simulink model "UNIFIER"  (R2023b)
settings: Solver=ode1  StartTime=0.0  StopTime=60  FixedStep=1/500  RelTol=1e-3
values from neighbouring files (symbols this model uses):
  b = 20.11467    [UNIFIER_LOAD.m]
  c = 1.43676    [UNIFIER_LOAD.m]
  DEP_INTEG_IC = 117.49388    [UNIFIER_LOAD.m]
  Euler0 = [3.43106170068520e-06, 0.0515008506277664, -2.79252663434261]    [UNIFIER_LOAD.m]
  ground_alt = 0    [UNIFIER_LOAD.m]
  h_ref_for_xplane = 0    [UNIFIER_LOAD.m]
  m = 7057    [UNIFIER_LOAD.m]
  omegab0 = [0,0,0]    [UNIFIER_LOAD.m]
  S = 29.98388    [UNIFIER_LOAD.m]
  sensor_delay_steps = 5    [UNIFIER_LOAD.m]
  u1_0 = [2.1112539e-05, -2.1112539e-05, -0.085004635, -0.084972650, 0.19720161, 0.19720161]    [UNIFIER_LOAD.m]
  u2_0 = ones(1,12) .* 0.4252    [UNIFIER_LOAD.m]
  u3_0 = 0.089689    [UNIFIER_LOAD.m]
  u4_0 = 0    [UNIFIER_LOAD.m]
  Vb0 = [52.6789583501891, 0, 2.71559652634250]    [UNIFIER_LOAD.m]
  vtail_dist_to_wing = 7.8070    (= 7.807)    [UNIFIER_LOAD.m]
  vtail_nodes = [dp_VTAIL.Xs_LE;     dp_VTAIL.Ys_LE;     dp_VTAIL.Zs_LE]    [UNIFIER_LOAD.m]
  wing_nodes = [fliplr(dp_WING_tip.LE_Xs),fliplr(dp_WING_root.LE_Xs),dp_WING_root.LE_Xs,dp_WING_tip.LE_Xs;     fliplr(-dp_WING_tip.LE_Ys),fliplr(-dp_WING_root.LE_Ys),dp_WING_root.LE_Ys,dp_WING_tip.LE_Ys;     fliplr(dp_WING_tip.LE_Zs),fliplr(dp_WING_root.LE_Zs),dp_WING_root.LE_Zs,dp_WING_tip.LE_Zs]    [UNIFIER_LOAD.m]
  Xe0 = [0,0,-1100]    [UNIFIER_LOAD.m]
  xyz_cg = [-8.09,0,-0.2]    [UNIFIER_LOAD.m]
  xyz_DEP = [ -6.9629998	-6.9210000	-6.8660002	-6.8099999	-6.7540002	-6.6999998	-6.6999998	-6.7540002	-6.8099999	-6.8660002	-6.9210000	-6.9629998 ... (first row only)    [UNIFIER_LOAD.m]
undefined symbols (not defined in the file or in its folder): dp_DEP, dp_FUSE_FIN, dp_HTU, dp_VTAIL, dp_VTAIL_INDUCED, dp_WING_root, dp_WING_tip, Earth, F, fcc, MIL, WGS84
libraries: aerolibactuator x16, dspnetwork x15, sharedutil x14, simulink_extras x13, sharedtransform x7, aerolibtransform2 x5, simulink x5, aerolibwind2 x4, matrix_library x1, shared6dof x1, aerolibatmos2 x1, slpidlib x1
(part 4 of 4)

== system UNIFIER/C7A_HARW/Subsystems/LandingGears/LeftMain/DetermineGroundImpact ==
  X_gear : Inport
  ground_alt : Inport  Port=2
  MATLAB Function : MATLAB Function  TreatAsAtomicUnit=on
  Memory : Memory  InitialCondition=[0,0,0]
  impactDetection : Subsystem
  dz_to_ground : Outport
  impact_flag : Outport  Port=2
  X_impact : Outport  Port=3
  wires:
  X_gear/1 -> MATLAB Function/1(X_tip_in), impactDetection/1(X_tip)
  ground_alt/1 -> impactDetection/2(ground_alt)
  MATLAB Function/1(X_tip_out) -> X_impact/1
  impactDetection/1(impact_flag) -> impact_flag/1, MATLAB Function/2(impact_flag)
  impactDetection/2(distance_to_ground) -> dz_to_ground/1
  MATLAB Function/2(X_tip_memory) -> Memory/1
  Memory/1 -> MATLAB Function/3("X_tip_memory ")

== system UNIFIER/C7A_HARW/Subsystems/LandingGears/LeftMain/FrameTransfer ==
  xyz_shock_absorber : Inport
  F_gear_total : Inport  Port=2
  Constant : Constant  Value=xyz_cg
  Sum : Sum  Inputs=+-
  cross product : sharedutil/3x3 Cross Product  aMode=aMode
  F_b : Outport
  M_b : Outport  Port=2
  wires:
  Sum/1 -> cross product/1
  xyz_shock_absorber/1 -> Sum/1
  Constant/1 -> Sum/2
  cross product/1 -> M_b/1
  F_gear_total/1 -> cross product/2, F_b/1  "F"

== system UNIFIER/C7A_HARW/Subsystems/LandingGears/LeftMain/GearForceSystem ==
  V_gear : Inport
  dz : Inport  Port=2
  impact_flag : Inport  Port=3  OutDataTypeStr=boolean
  Constant : Constant  Value=0
  Demux : Demux  Outputs=3
  Forcez : Subsystem
  Mux : Mux  Inputs=3
  Terminator1 : Terminator
  Terminator2 : Terminator
  Unary Minus : UnaryMinus
  groundContactLogic3 : Subsystem
  F_gear_total : Outport
  wires:
  dz/1 -> groundContactLogic3/1(in)
  Forcez/1(Fz) -> Mux/3
  impact_flag/1 -> groundContactLogic3/3(flag)
  groundContactLogic3/1(out) -> Forcez/1(d)
  groundContactLogic3/2(out_dt) -> Forcez/2(d_dt)
  Demux/3 -> groundContactLogic3/2(in_dt)
  V_gear/1 -> Unary Minus/1
  Mux/1 -> F_gear_total/1
  Demux/1 -> Terminator1/1
  Unary Minus/1 -> Demux/1
  Constant/1 -> Mux/2, Mux/1
  Demux/2 -> Terminator2/1

== system UNIFIER/C7A_HARW/Subsystems/LandingGears/LeftMain/GetDeflection ==
  X_impact : Inport
  X_tip : Inport  Port=2
  Demux : Demux  Outputs=3
  Sum1 : Sum  Inputs=|+-
  Terminator : Terminator
  Terminator1 : Terminator
  dz : Outport
  wires:
  X_impact/1 -> Sum1/1
  X_tip/1 -> Sum1/2
  Demux/1 -> Terminator1/1
  Demux/3 -> dz/1
  Sum1/1 -> Demux/1
  Demux/2 -> Terminator/1

== system UNIFIER/C7A_HARW/Subsystems/LandingGears/LeftMain/PointAndVelocityTransformation ==
  xyz_gear : Inport
  X_e : Inport  Port=2
  Euler : Inport  Port=3
  omega : Inport  Port=4
  V_b : Inport  Port=5
  Constant : Constant  Value=xyz_cg
  Constant1 : Constant  Value=0
  Demux1 : Demux  Outputs=3
  Demux3 : Demux  Outputs=3
  Mux : Mux  Inputs=3
  Mux2 : Mux  Inputs=3
  Product : Product  Multiplication=Matrix(*)
  Product1 : Product  Multiplication=Matrix(*)
  Rotation Angles to Direction Cosine Matrix : sharedtransform/Rotation Angles to Direction Cosine Matrix  rotationOrder=ZYX  aMode=aMode
  Rotation Angles to Direction Cosine Matrix1 : sharedtransform/Rotation Angles to Direction Cosine Matrix  rotationOrder=ZYX  aMode=aMode
  Sum : Sum  Inputs=+-
  Sum1 : Sum  Inputs=++|
  Sum3 : Sum  Inputs=++|
  Terminator : Terminator
  Transpose : Math  Operator=transpose
  Transpose1 : Math  Operator=transpose
  cross product1 : sharedutil/3x3 Cross Product  aMode=aMode
  X_gear : Outport
  V_gear : Outport  Port=2
  wires:
  Sum1/1 -> X_gear/1
  Constant/1 -> Sum/2
  X_e/1 -> Sum1/1
  xyz_gear/1 -> Sum/1
  cross product1/1 -> Sum3/1
  Sum/1 -> Product/2, cross product1/2
  Product/1 -> Sum1/2
  Rotation Angles to Direction Cosine Matrix/1 -> Transpose/1
  Transpose/1 -> Product/1
  Demux3/2 -> Mux/2
  Demux3/1 -> Mux/3
  Mux/1 -> Rotation Angles to Direction Cosine Matrix/1
  omega/1 -> cross product1/1
  V_b/1 -> Sum3/2
  Sum3/1 -> Product1/2
  Demux3/3 -> Mux/1
  Product1/1 -> V_gear/1
  Demux1/1 -> Mux2/3
  Rotation Angles to Direction Cosine Matrix1/1 -> Transpose1/1
  Demux1/2 -> Mux2/2
  Mux2/1 -> Rotation Angles to Direction Cosine Matrix1/1
  Transpose1/1 -> Product1/1
  Constant1/1 -> Mux2/1
  Demux1/3 -> Terminator/1
  Euler/1 -> Demux1/1, Demux3/1

== system UNIFIER/C7A_HARW/Subsystems/LandingGears/Nose/DetermineGroundImpact ==
  X_gear : Inport
  ground_alt : Inport  Port=2
  MATLAB Function : MATLAB Function  TreatAsAtomicUnit=on
  Memory : Memory  InitialCondition=[0,0,0]
  impactDetection : Subsystem
  dz_to_ground : Outport
  impact_flag : Outport  Port=2
  X_impact : Outport  Port=3
  wires:
  X_gear/1 -> MATLAB Function/1(X_tip_in), impactDetection/1(X_tip)
  ground_alt/1 -> impactDetection/2(ground_alt)
  MATLAB Function/1(X_tip_out) -> X_impact/1
  impactDetection/1(impact_flag) -> impact_flag/1, MATLAB Function/2(impact_flag)
  impactDetection/2(distance_to_ground) -> dz_to_ground/1
  MATLAB Function/2(X_tip_memory) -> Memory/1
  Memory/1 -> MATLAB Function/3("X_tip_memory ")

== system UNIFIER/C7A_HARW/Subsystems/LandingGears/Nose/FrameTransfer ==
  xyz_shock_absorber : Inport
  F_gear_total : Inport  Port=2
  Constant : Constant  Value=xyz_cg
  Sum : Sum  Inputs=+-
  cross product : sharedutil/3x3 Cross Product  aMode=aMode
  F_b : Outport
  M_b : Outport  Port=2
  wires:
  Sum/1 -> cross product/1
  xyz_shock_absorber/1 -> Sum/1
  Constant/1 -> Sum/2
  cross product/1 -> M_b/1
  F_gear_total/1 -> cross product/2, F_b/1  "F"

== system UNIFIER/C7A_HARW/Subsystems/LandingGears/Nose/GearForceSystem ==
  V_gear : Inport
  dz : Inport  Port=2
  impact_flag : Inport  Port=3  OutDataTypeStr=boolean
  Constant : Constant  Value=0
  Demux : Demux  Outputs=3
  Forcez : Subsystem
  Mux : Mux  Inputs=3
  Terminator1 : Terminator
  Terminator2 : Terminator
  Unary Minus : UnaryMinus
  groundContactLogic3 : Subsystem
  F_gear_total : Outport
  wires:
  dz/1 -> groundContactLogic3/1(in)
  Forcez/1(Fz) -> Mux/3
  impact_flag/1 -> groundContactLogic3/3(flag)
  groundContactLogic3/1(out) -> Forcez/1(d)
  groundContactLogic3/2(out_dt) -> Forcez/2(d_dt)
  Demux/3 -> groundContactLogic3/2(in_dt)
  V_gear/1 -> Unary Minus/1
  Mux/1 -> F_gear_total/1
  Demux/1 -> Terminator1/1
  Unary Minus/1 -> Demux/1
  Constant/1 -> Mux/2, Mux/1
  Demux/2 -> Terminator2/1

== system UNIFIER/C7A_HARW/Subsystems/LandingGears/Nose/GetDeflection ==
  X_impact : Inport
  X_tip : Inport  Port=2
  Demux : Demux  Outputs=3
  Sum1 : Sum  Inputs=|+-
  Terminator : Terminator
  Terminator1 : Terminator
  dz : Outport
  wires:
  X_impact/1 -> Sum1/1
  X_tip/1 -> Sum1/2
  Demux/1 -> Terminator1/1
  Demux/3 -> dz/1
  Sum1/1 -> Demux/1
  Demux/2 -> Terminator/1

== system UNIFIER/C7A_HARW/Subsystems/LandingGears/Nose/PointAndVelocityTransformation ==
  xyz_gear : Inport
  X_e : Inport  Port=2
  Euler : Inport  Port=3
  omega : Inport  Port=4
  V_b : Inport  Port=5
  Constant : Constant  Value=xyz_cg
  Constant1 : Constant  Value=0
  Demux1 : Demux  Outputs=3
  Demux3 : Demux  Outputs=3
  Mux : Mux  Inputs=3
  Mux2 : Mux  Inputs=3
  Product : Product  Multiplication=Matrix(*)
  Product1 : Product  Multiplication=Matrix(*)
  Rotation Angles to Direction Cosine Matrix : sharedtransform/Rotation Angles to Direction Cosine Matrix  rotationOrder=ZYX  aMode=aMode
  Rotation Angles to Direction Cosine Matrix1 : sharedtransform/Rotation Angles to Direction Cosine Matrix  rotationOrder=ZYX  aMode=aMode
  Sum : Sum  Inputs=+-
  Sum1 : Sum  Inputs=++|
  Sum3 : Sum  Inputs=++|
  Terminator : Terminator
  Transpose : Math  Operator=transpose
  Transpose1 : Math  Operator=transpose
  cross product1 : sharedutil/3x3 Cross Product  aMode=aMode
  X_gear : Outport
  V_gear : Outport  Port=2
  wires:
  Sum1/1 -> X_gear/1
  Constant/1 -> Sum/2
  X_e/1 -> Sum1/1
  xyz_gear/1 -> Sum/1
  cross product1/1 -> Sum3/1
  Sum/1 -> Product/2, cross product1/2
  Product/1 -> Sum1/2
  Rotation Angles to Direction Cosine Matrix/1 -> Transpose/1
  Transpose/1 -> Product/1
  Demux3/2 -> Mux/2
  Demux3/1 -> Mux/3
  Mux/1 -> Rotation Angles to Direction Cosine Matrix/1
  omega/1 -> cross product1/1
  V_b/1 -> Sum3/2
  Sum3/1 -> Product1/2
  Demux3/3 -> Mux/1
  Product1/1 -> V_gear/1
  Demux1/1 -> Mux2/3
  Rotation Angles to Direction Cosine Matrix1/1 -> Transpose1/1
  Demux1/2 -> Mux2/2
  Mux2/1 -> Rotation Angles to Direction Cosine Matrix1/1
  Transpose1/1 -> Product1/1
  Constant1/1 -> Mux2/1
  Demux1/3 -> Terminator/1
  Euler/1 -> Demux1/1, Demux3/1

== system UNIFIER/C7A_HARW/Subsystems/LandingGears/RightMain/DetermineGroundImpact ==
  X_gear : Inport
  ground_alt : Inport  Port=2
  MATLAB Function : MATLAB Function  TreatAsAtomicUnit=on
  Memory : Memory  InitialCondition=[0,0,0]
  impactDetection : Subsystem
  dz_to_ground : Outport
  impact_flag : Outport  Port=2
  X_impact : Outport  Port=3
  wires:
  X_gear/1 -> MATLAB Function/1(X_tip_in), impactDetection/1(X_tip)
  ground_alt/1 -> impactDetection/2(ground_alt)
  MATLAB Function/1(X_tip_out) -> X_impact/1
  impactDetection/1(impact_flag) -> impact_flag/1, MATLAB Function/2(impact_flag)
  impactDetection/2(distance_to_ground) -> dz_to_ground/1
  MATLAB Function/2(X_tip_memory) -> Memory/1
  Memory/1 -> MATLAB Function/3("X_tip_memory ")

== system UNIFIER/C7A_HARW/Subsystems/LandingGears/RightMain/FrameTransfer ==
  xyz_shock_absorber : Inport
  F_gear_total : Inport  Port=2
  Constant : Constant  Value=xyz_cg
  Sum : Sum  Inputs=+-
  cross product : sharedutil/3x3 Cross Product  aMode=aMode
  F_b : Outport
  M_b : Outport  Port=2
  wires:
  Sum/1 -> cross product/1
  xyz_shock_absorber/1 -> Sum/1
  Constant/1 -> Sum/2
  cross product/1 -> M_b/1
  F_gear_total/1 -> cross product/2, F_b/1  "F"

== system UNIFIER/C7A_HARW/Subsystems/LandingGears/RightMain/GearForceSystem ==
  V_gear : Inport
  dz : Inport  Port=2
  impact_flag : Inport  Port=3  OutDataTypeStr=boolean
  Constant : Constant  Value=0
  Demux : Demux  Outputs=3
  Forcez : Subsystem
  Mux : Mux  Inputs=3
  Terminator1 : Terminator
  Terminator2 : Terminator
  Unary Minus : UnaryMinus
  groundContactLogic3 : Subsystem
  F_gear_total : Outport
  wires:
  dz/1 -> groundContactLogic3/1(in)
  Forcez/1(Fz) -> Mux/3
  impact_flag/1 -> groundContactLogic3/3(flag)
  groundContactLogic3/1(out) -> Forcez/1(d)
  groundContactLogic3/2(out_dt) -> Forcez/2(d_dt)
  Demux/3 -> groundContactLogic3/2(in_dt)
  V_gear/1 -> Unary Minus/1
  Mux/1 -> F_gear_total/1
  Demux/1 -> Terminator1/1
  Unary Minus/1 -> Demux/1
  Constant/1 -> Mux/2, Mux/1
  Demux/2 -> Terminator2/1

== system UNIFIER/C7A_HARW/Subsystems/LandingGears/RightMain/GetDeflection ==
  X_impact : Inport
  X_tip : Inport  Port=2
  Demux : Demux  Outputs=3
  Sum1 : Sum  Inputs=|+-
  Terminator : Terminator
  Terminator1 : Terminator
  dz : Outport
  wires:
  X_impact/1 -> Sum1/1
  X_tip/1 -> Sum1/2
  Demux/1 -> Terminator1/1
  Demux/3 -> dz/1
  Sum1/1 -> Demux/1
  Demux/2 -> Terminator/1

== system UNIFIER/C7A_HARW/Subsystems/LandingGears/RightMain/PointAndVelocityTransformation ==
  xyz_gear : Inport
  X_e : Inport  Port=2
  Euler : Inport  Port=3
  omega : Inport  Port=4
  V_b : Inport  Port=5
  Constant : Constant  Value=xyz_cg
  Constant1 : Constant  Value=0
  Demux1 : Demux  Outputs=3
  Demux3 : Demux  Outputs=3
  Mux : Mux  Inputs=3
  Mux2 : Mux  Inputs=3
  Product : Product  Multiplication=Matrix(*)
  Product1 : Product  Multiplication=Matrix(*)
  Rotation Angles to Direction Cosine Matrix : sharedtransform/Rotation Angles to Direction Cosine Matrix  rotationOrder=ZYX  aMode=aMode
  Rotation Angles to Direction Cosine Matrix1 : sharedtransform/Rotation Angles to Direction Cosine Matrix  rotationOrder=ZYX  aMode=aMode
  Sum : Sum  Inputs=+-
  Sum1 : Sum  Inputs=++|
  Sum3 : Sum  Inputs=++|
  Terminator : Terminator
  Transpose : Math  Operator=transpose
  Transpose1 : Math  Operator=transpose
  cross product1 : sharedutil/3x3 Cross Product  aMode=aMode
  X_gear : Outport
  V_gear : Outport  Port=2
  wires:
  Sum1/1 -> X_gear/1
  Constant/1 -> Sum/2
  X_e/1 -> Sum1/1
  xyz_gear/1 -> Sum/1
  cross product1/1 -> Sum3/1
  Sum/1 -> Product/2, cross product1/2
  Product/1 -> Sum1/2
  Rotation Angles to Direction Cosine Matrix/1 -> Transpose/1
  Transpose/1 -> Product/1
  Demux3/2 -> Mux/2
  Demux3/1 -> Mux/3
  Mux/1 -> Rotation Angles to Direction Cosine Matrix/1
  omega/1 -> cross product1/1
  V_b/1 -> Sum3/2
  Sum3/1 -> Product1/2
  Demux3/3 -> Mux/1
  Product1/1 -> V_gear/1
  Demux1/1 -> Mux2/3
  Rotation Angles to Direction Cosine Matrix1/1 -> Transpose1/1
  Demux1/2 -> Mux2/2
  Mux2/1 -> Rotation Angles to Direction Cosine Matrix1/1
  Transpose1/1 -> Product1/1
  Constant1/1 -> Mux2/1
  Demux1/3 -> Terminator/1
  Euler/1 -> Demux1/1, Demux3/1

== system UNIFIER/C7A_HARW/Subsystems/LandingGears/SideForceAndSteeringAndBraking/ForceSystem ==
  impact_flag_main : Inport  OutDataTypeStr=boolean
  impact_flag_nose : Inport  Port=2  OutDataTypeStr=boolean
  V_b : Inport  Port=3
  Fz_main : Inport  Port=4
  Fz_nose : Inport  Port=5
  yaw_raw : Inport  Port=6
  buttons : Inport  Port=7
  Constant2 : Constant  Value=0
  Constant3 : Constant  Value=0
  Demux : Demux  Outputs=3
  MainGearBrake : Subsystem
  MainGearSideForce : Subsystem
  Mux : Mux  Inputs=3
  Mux1 : Mux  Inputs=3
  NoseWheelSteer : Subsystem
  Scope : Scope
  Selector : Selector  InputPortWidth=12  IndexOptions=Index vector (dialog)  Indices=1  OutputSizes=1
  Terminator1 : Terminator
  Terminator2 : Terminator
  Unary Minus : UnaryMinus
  groundContactLogic3 : Subsystem
  F_main_gear : Outport
  F_nose_gear : Outport  Port=2
  wires:
  impact_flag_main/1 -> groundContactLogic3/2(flag)
  groundContactLogic3/1(out_dt) -> MainGearSideForce/1(d_dt)
  Demux/2 -> groundContactLogic3/1(in_dt)
  V_b/1 -> Unary Minus/1
  Mux/1 -> F_main_gear/1
  Demux/1 -> Terminator1/1
  Unary Minus/1 -> Demux/1
  Demux/3 -> Terminator2/1
  MainGearBrake/1(Fx) -> Mux/1
  buttons/1 -> Selector/1
  Selector/1 -> Scope/1, MainGearBrake/1(brake)
  Fz_main/1 -> MainGearBrake/2(Fz_main), MainGearSideForce/2(Fz_main)
  MainGearSideForce/1(Fy) -> Mux/2
  Constant2/1 -> Mux/3
  Mux1/1 -> F_nose_gear/1
  Constant3/1 -> Mux1/3, Mux1/1
  yaw_raw/1 -> NoseWheelSteer/1(yaw_raw)
  impact_flag_nose/1 -> NoseWheelSteer/2(impact_flag_nose)
  Fz_nose/1 -> NoseWheelSteer/3(Fz_nose)
  NoseWheelSteer/1(y) -> Mux1/2

== system UNIFIER/C7A_HARW/Subsystems/LandingGears/SideForceAndSteeringAndBraking/FrameTransfer1 ==
  xyz : Inport
  F_total : Inport  Port=2
  Constant : Constant  Value=xyz_cg
  Sum : Sum  Inputs=+-
  cross product : sharedutil/3x3 Cross Product  aMode=aMode
  F_b : Outport
  M_b : Outport  Port=2
  wires:
  Sum/1 -> cross product/1
  xyz/1 -> Sum/1
  Constant/1 -> Sum/2
  cross product/1 -> M_b/1
  F_total/1 -> cross product/2, F_b/1  "F"

== system UNIFIER/C7A_HARW/Subsystems/LandingGears/SideForceAndSteeringAndBraking/FrameTransfer2 ==
  xyz : Inport
  F_total : Inport  Port=2
  Constant : Constant  Value=xyz_cg
  Sum : Sum  Inputs=+-
  cross product : sharedutil/3x3 Cross Product  aMode=aMode
  F_b : Outport
  M_b : Outport  Port=2
  wires:
  F_total/1 -> F_b/1, cross product/2  "F"
  cross product/1 -> M_b/1
  Constant/1 -> Sum/2
  xyz/1 -> Sum/1
  Sum/1 -> cross product/1

== system UNIFIER/C7A_HARW/Aero/WingForces/Left/Subsystem/CrossProduct ==
  r : Inport  Partition=on  PartitionDimension=2  PartitionWidth=1  PartitionOffset=0
  F : Inport  Port=2  Partition=on  PartitionDimension=2  PartitionWidth=1  PartitionOffset=0
  3x3 Cross Product : sharedutil/3x3 Cross Product  aMode=aMode
  CG : Constant  Value=xyz_cg
  Cast : DataTypeConversion  OutDataTypeStr=single  SaturateOnIntegerOverflow=off  RndMeth=Floor
  For Each : ForEach  DisableCoverage=on  SpecifiedNumIters=7
  Minus : Sum  Inputs=+-
  M : Outport  ConcatenationDimension=2
  wires:
  F/1 -> 3x3 Cross Product/2
  r/1 -> Minus/1
  3x3 Cross Product/1 -> M/1
  CG/1 -> Cast/1
  Minus/1 -> 3x3 Cross Product/1
  Cast/1 -> Minus/2

== system UNIFIER/C7A_HARW/Aero/WingForces/Left/Subsystem/w2b ==
  alpha : Inport  OutDataTypeStr=single  Partition=on  PartitionDimension=1  PartitionWidth=1  PartitionOffset=0
  Fw : Inport  Port=2  Partition=on  PartitionDimension=2  PartitionWidth=1  PartitionOffset=0
  Cast To Double : DataTypeConversion  OutDataTypeStr=double  SaturateOnIntegerOverflow=off  RndMeth=Floor
  Cast To Single : DataTypeConversion  OutDataTypeStr=single  SaturateOnIntegerOverflow=off  RndMeth=Floor
  Constant : Constant  Value=0  OutDataTypeStr=single
  Demux : Demux  Outputs=3
  Direction Cosine Matrix Body to Wind : aerolibtransform2/Direction Cosine Matrix Body to Wind
  Display : Display
  Display1 : Display
  For Each : ForEach  DisableCoverage=on  SpecifiedNumIters=7
  Matrix Multiply : Product  Multiplication=Matrix(*)
  Mux : Mux  Inputs=3
  Mux1 : Mux  Inputs=2
  Transpose : Math  Operator=transpose
  Unary Minus : UnaryMinus
  Unary Minus1 : UnaryMinus
  Fb : Outport  ConcatenationDimension=2
  wires:
  Fw/1 -> Display1/1, Demux/1
  alpha/1 -> Display/1, Mux1/1
  Matrix Multiply/1 -> Fb/1
  Mux/1 -> Matrix Multiply/2
  Demux/1 -> Unary Minus/1
  Unary Minus/1 -> Mux/1
  Demux/2 -> Mux/2
  Unary Minus1/1 -> Mux/3
  Demux/3 -> Unary Minus1/1
  Direction Cosine Matrix Body to Wind/1 -> Transpose/1
  Transpose/1 -> Cast To Single/1
  Mux1/1 -> Cast To Double/1
  Constant/1 -> Mux1/2
  Cast To Single/1 -> Matrix Multiply/1
  Cast To Double/1 -> Direction Cosine Matrix Body to Wind/1

== system UNIFIER/C7A_HARW/Aero/WingForces/Left/WingRootForces/WingRootPreLookup ==
  flap_defl : Inport
  alpha : Inport  Port=2
  V_node : Inport  Port=3
  DEP_J : Inport  Port=4
  Constant8 : Constant  Value=0:4
  Prelookup : PreLookup  BreakpointsData=dp_WING_root.flap_defl  IndexSearchMethod=Linear search  BeginIndexSearchUsingPreviousIndexResult=on  UseLastBreakpoint=on
  Prelookup1 : PreLookup  BreakpointsData=dp_WING_root.alphas  IndexSearchMethod=Linear search  BeginIndexSearchUsingPreviousIndexResult=on  UseLastBreakpoint=on
  Prelookup2 : PreLookup  BreakpointsData=dp_WING_root.V  IndexSearchMethod=Linear search  BeginIndexSearchUsingPreviousIndexResult=on  UseLastBreakpoint=on
  Prelookup3 : PreLookup  BreakpointsData=dp_WING_root.DEP_J  IndexSearchMethod=Linear search  BeginIndexSearchUsingPreviousIndexResult=on  UseLastBreakpoint=on
  Out1 : Outport
  Out2 : Outport  Port=2
  Out3 : Outport  Port=3
  Out4 : Outport  Port=4
  Out6 : Outport  Port=5
  Out7 : Outport  Port=6
  Out8 : Outport  Port=7
  Out9 : Outport  Port=8
  Out5 : Outport  Port=9
  wires:
  Prelookup/1 -> Out1/1
  Constant8/1 -> Out5/1
  Prelookup1/2 -> Out4/1
  Prelookup/2 -> Out2/1
  alpha/1 -> Prelookup1/1
  Prelookup1/1 -> Out3/1
  flap_defl/1 -> Prelookup/1
  V_node/1 -> Prelookup2/1
  DEP_J/1 -> Prelookup3/1
  Prelookup2/1 -> Out6/1
  Prelookup2/2 -> Out7/1
  Prelookup3/1 -> Out8/1
  Prelookup3/2 -> Out9/1

== system UNIFIER/C7A_HARW/Aero/WingForces/Left/WingTipForces/WingRootPreLookup ==
  ail_defl : Inport
  alpha : Inport  Port=2
  V_node : Inport  Port=3
  DEP_J : Inport  Port=4
  Constant8 : Constant  Value=0:1
  Prelookup : PreLookup  BreakpointsData=dp_WING_tip.ail_defl  IndexSearchMethod=Linear search  BeginIndexSearchUsingPreviousIndexResult=on  UseLastBreakpoint=on
  Prelookup1 : PreLookup  BreakpointsData=dp_WING_tip.alphas  IndexSearchMethod=Linear search  BeginIndexSearchUsingPreviousIndexResult=on  UseLastBreakpoint=on
  Prelookup2 : PreLookup  BreakpointsData=dp_WING_tip.V  IndexSearchMethod=Linear search  BeginIndexSearchUsingPreviousIndexResult=on  UseLastBreakpoint=on
  Prelookup3 : PreLookup  BreakpointsData=dp_WING_tip.DEP_J  IndexSearchMethod=Linear search  BeginIndexSearchUsingPreviousIndexResult=on  UseLastBreakpoint=on
  Out1 : Outport
  Out2 : Outport  Port=2
  Out3 : Outport  Port=3
  Out4 : Outport  Port=4
  Out6 : Outport  Port=5
  Out7 : Outport  Port=6
  Out8 : Outport  Port=7
  Out9 : Outport  Port=8
  Out5 : Outport  Port=9
  wires:
  Prelookup/1 -> Out1/1
  Constant8/1 -> Out5/1
  Prelookup1/2 -> Out4/1
  Prelookup/2 -> Out2/1
  alpha/1 -> Prelookup1/1
  Prelookup1/1 -> Out3/1
  ail_defl/1 -> Prelookup/1
  V_node/1 -> Prelookup2/1
  DEP_J/1 -> Prelookup3/1
  Prelookup2/1 -> Out6/1
  Prelookup2/2 -> Out7/1
  Prelookup3/1 -> Out8/1
  Prelookup3/2 -> Out9/1

== system UNIFIER/C7A_HARW/Aero/WingForces/Right/Subsystem/CrossProduct ==
  r : Inport  Partition=on  PartitionDimension=2  PartitionWidth=1  PartitionOffset=0
  F : Inport  Port=2  Partition=on  PartitionDimension=2  PartitionWidth=1  PartitionOffset=0
  3x3 Cross Product : sharedutil/3x3 Cross Product  aMode=aMode
  CG : Constant  Value=xyz_cg
  Cast : DataTypeConversion  OutDataTypeStr=single  SaturateOnIntegerOverflow=off  RndMeth=Floor
  For Each : ForEach  DisableCoverage=on  SpecifiedNumIters=7
  Minus : Sum  Inputs=+-
  M : Outport  ConcatenationDimension=2
  wires:
  F/1 -> 3x3 Cross Product/2
  r/1 -> Minus/1
  3x3 Cross Product/1 -> M/1
  CG/1 -> Cast/1
  Minus/1 -> 3x3 Cross Product/1
  Cast/1 -> Minus/2

== system UNIFIER/C7A_HARW/Aero/WingForces/Right/Subsystem/w2b ==
  alpha : Inport  OutDataTypeStr=single  Partition=on  PartitionDimension=1  PartitionWidth=1  PartitionOffset=0
  Fw : Inport  Port=2  Partition=on  PartitionDimension=2  PartitionWidth=1  PartitionOffset=0
  Cast To Double : DataTypeConversion  OutDataTypeStr=double  SaturateOnIntegerOverflow=off  RndMeth=Floor
  Cast To Single : DataTypeConversion  OutDataTypeStr=single  SaturateOnIntegerOverflow=off  RndMeth=Floor
  Constant : Constant  Value=0  OutDataTypeStr=single
  Demux : Demux  Outputs=3
  Direction Cosine Matrix Body to Wind : aerolibtransform2/Direction Cosine Matrix Body to Wind
  Display : Display
  Display1 : Display
  For Each : ForEach  DisableCoverage=on  SpecifiedNumIters=7
  Matrix Multiply : Product  Multiplication=Matrix(*)
  Mux : Mux  Inputs=3
  Mux1 : Mux  Inputs=2
  Transpose : Math  Operator=transpose
  Unary Minus : UnaryMinus
  Unary Minus1 : UnaryMinus
  Fb : Outport  ConcatenationDimension=2
  wires:
  Fw/1 -> Display1/1, Demux/1
  alpha/1 -> Display/1, Mux1/1
  Matrix Multiply/1 -> Fb/1
  Mux/1 -> Matrix Multiply/2
  Demux/1 -> Unary Minus/1
  Unary Minus/1 -> Mux/1
  Demux/2 -> Mux/2
  Unary Minus1/1 -> Mux/3
  Demux/3 -> Unary Minus1/1
  Direction Cosine Matrix Body to Wind/1 -> Transpose/1
  Transpose/1 -> Cast To Single/1
  Mux1/1 -> Cast To Double/1
  Constant/1 -> Mux1/2
  Cast To Single/1 -> Matrix Multiply/1
  Cast To Double/1 -> Direction Cosine Matrix Body to Wind/1

== system UNIFIER/C7A_HARW/Aero/WingForces/Right/WingRootForces/WingRootPreLookup ==
  flap_defl : Inport
  alpha : Inport  Port=2
  V_node : Inport  Port=3
  DEP_J : Inport  Port=4
  Constant8 : Constant  Value=0:4
  Prelookup : PreLookup  BreakpointsData=dp_WING_root.flap_defl  IndexSearchMethod=Linear search  BeginIndexSearchUsingPreviousIndexResult=on  UseLastBreakpoint=on
  Prelookup1 : PreLookup  BreakpointsData=dp_WING_root.alphas  IndexSearchMethod=Linear search  BeginIndexSearchUsingPreviousIndexResult=on  UseLastBreakpoint=on
  Prelookup2 : PreLookup  BreakpointsData=dp_WING_root.V  IndexSearchMethod=Linear search  BeginIndexSearchUsingPreviousIndexResult=on  UseLastBreakpoint=on
  Prelookup3 : PreLookup  BreakpointsData=dp_WING_root.DEP_J  IndexSearchMethod=Linear search  BeginIndexSearchUsingPreviousIndexResult=on  UseLastBreakpoint=on
  Out1 : Outport
  Out2 : Outport  Port=2
  Out3 : Outport  Port=3
  Out4 : Outport  Port=4
  Out6 : Outport  Port=5
  Out7 : Outport  Port=6
  Out8 : Outport  Port=7
  Out9 : Outport  Port=8
  Out5 : Outport  Port=9
  wires:
  Prelookup/1 -> Out1/1
  Constant8/1 -> Out5/1
  Prelookup1/2 -> Out4/1
  Prelookup/2 -> Out2/1
  alpha/1 -> Prelookup1/1
  Prelookup1/1 -> Out3/1
  flap_defl/1 -> Prelookup/1
  V_node/1 -> Prelookup2/1
  DEP_J/1 -> Prelookup3/1
  Prelookup2/1 -> Out6/1
  Prelookup2/2 -> Out7/1
  Prelookup3/1 -> Out8/1
  Prelookup3/2 -> Out9/1

== system UNIFIER/C7A_HARW/Aero/WingForces/Right/WingTipForces/WingRootPreLookup ==
  ail_defl : Inport
  alpha : Inport  Port=2
  V_node : Inport  Port=3
  DEP_J : Inport  Port=4
  Constant8 : Constant  Value=0:1
  Prelookup : PreLookup  BreakpointsData=dp_WING_tip.ail_defl  IndexSearchMethod=Linear search  BeginIndexSearchUsingPreviousIndexResult=on  UseLastBreakpoint=on
  Prelookup1 : PreLookup  BreakpointsData=dp_WING_tip.alphas  IndexSearchMethod=Linear search  BeginIndexSearchUsingPreviousIndexResult=on  UseLastBreakpoint=on
  Prelookup2 : PreLookup  BreakpointsData=dp_WING_tip.V  IndexSearchMethod=Linear search  BeginIndexSearchUsingPreviousIndexResult=on  UseLastBreakpoint=on
  Prelookup3 : PreLookup  BreakpointsData=dp_WING_tip.DEP_J  IndexSearchMethod=Linear search  BeginIndexSearchUsingPreviousIndexResult=on  UseLastBreakpoint=on
  Out1 : Outport
  Out2 : Outport  Port=2
  Out3 : Outport  Port=3
  Out4 : Outport  Port=4
  Out6 : Outport  Port=5
  Out7 : Outport  Port=6
  Out8 : Outport  Port=7
  Out9 : Outport  Port=8
  Out5 : Outport  Port=9
  wires:
  Prelookup/1 -> Out1/1
  Constant8/1 -> Out5/1
  Prelookup1/2 -> Out4/1
  Prelookup/2 -> Out2/1
  alpha/1 -> Prelookup1/1
  Prelookup1/1 -> Out3/1
  ail_defl/1 -> Prelookup/1
  V_node/1 -> Prelookup2/1
  DEP_J/1 -> Prelookup3/1
  Prelookup2/1 -> Out6/1
  Prelookup2/2 -> Out7/1
  Prelookup3/1 -> Out8/1
  Prelookup3/2 -> Out9/1

== system UNIFIER/C7A_HARW/Subsystems/LandingGears/LeftMain/DetermineGroundImpact/impactDetection ==
  note: Impact
  note: No impact
  X_tip : Inport
  ground_alt : Inport  Port=2
  Constant : Constant  OutDataTypeStr=boolean
  Constant1 : Constant  Value=0  OutDataTypeStr=boolean
  Selector1 : Selector  InputPortWidth=3  IndexOptions=Index vector (dialog)  Indices=3  OutputSizes=1
  Sum : Sum  Inputs=-+|
  Switch : Switch  Criteria=u2 > Threshold  SaturateOnIntegerOverflow=off  InputSameDT=off
  impact_flag : Outport
  distance_to_ground : Outport  Port=2
  wires:
  Constant1/1 -> Switch/1
  ground_alt/1 -> Sum/2
  X_tip/1 -> Selector1/1
  Selector1/1 -> Sum/1
  Switch/1 -> impact_flag/1
  Constant/1 -> Switch/3
  Sum/1 -> distance_to_ground/1, Switch/2

== system UNIFIER/C7A_HARW/Subsystems/LandingGears/LeftMain/GearForceSystem/Forcez ==
  d : Inport
  d_dt : Inport  Port=2
  Constant : Constant  Value=110000
  Constant1 : Constant  Value=7000
  Constant2 : Constant  Value=0.15
  Product : Product
  Product1 : Product
  Saturation : Saturate  UpperLimit=0  LowerLimit=-inf
  Saturation1 : Saturate  UpperLimit=0  LowerLimit=-inf
  Scope : Scope  NumInputPorts=2
  Scope1 : Scope
  Sum : Sum  Inputs=|++
  Sum1 : Sum  Inputs=|++
  Fz : Outport
  wires:
  Constant1/1 -> Product1/1
  d_dt/1 -> Product1/2
  Constant/1 -> Product/2
  Product1/1 -> Scope/2, Sum/2
  d/1 -> Sum1/1
  Product/1 -> Scope/1, Sum/1
  Sum/1 -> Scope1/1, Saturation/1
  Saturation/1 -> Fz/1
  Sum1/1 -> Saturation1/1
  Constant2/1 -> Sum1/2
  Saturation1/1 -> Product/1

== system UNIFIER/C7A_HARW/Subsystems/LandingGears/LeftMain/GearForceSystem/groundContactLogic3 ==
  in : Inport
  in_dt : Inport  Port=2
  flag : Inport  Port=3  OutDataTypeStr=boolean
  Constant : Constant  Value=0
  Switch : Switch  Criteria=u2 ~= 0  SaturateOnIntegerOverflow=off  InputSameDT=off
  Switch1 : Switch  Criteria=u2 > Threshold  SaturateOnIntegerOverflow=off  InputSameDT=off
  out : Outport
  out_dt : Outport  Port=2
  wires:
  Switch1/1 -> out_dt/1
  Switch/1 -> out/1
  in/1 -> Switch/1
  in_dt/1 -> Switch1/1
  flag/1 -> Switch1/2, Switch/2
  Constant/1 -> Switch/3, Switch1/3

== system UNIFIER/C7A_HARW/Subsystems/LandingGears/Nose/DetermineGroundImpact/impactDetection ==
  note: Impact
  note: No impact
  X_tip : Inport
  ground_alt : Inport  Port=2
  Constant : Constant  OutDataTypeStr=boolean
  Constant1 : Constant  Value=0  OutDataTypeStr=boolean
  Selector1 : Selector  InputPortWidth=3  IndexOptions=Index vector (dialog)  Indices=3  OutputSizes=1
  Sum : Sum  Inputs=-+|
  Switch : Switch  Criteria=u2 > Threshold  SaturateOnIntegerOverflow=off  InputSameDT=off
  impact_flag : Outport
  distance_to_ground : Outport  Port=2
  wires:
  Constant1/1 -> Switch/1
  ground_alt/1 -> Sum/2
  X_tip/1 -> Selector1/1
  Selector1/1 -> Sum/1
  Switch/1 -> impact_flag/1
  Constant/1 -> Switch/3
  Sum/1 -> distance_to_ground/1, Switch/2

== system UNIFIER/C7A_HARW/Subsystems/LandingGears/Nose/GearForceSystem/Forcez ==
  d : Inport
  d_dt : Inport  Port=2
  Constant : Constant  Value=110000
  Constant1 : Constant  Value=7000
  Constant2 : Constant  Value=0.15
  Product : Product
  Product1 : Product
  Saturation : Saturate  UpperLimit=0  LowerLimit=-inf
  Saturation1 : Saturate  UpperLimit=0  LowerLimit=-inf
  Scope : Scope  NumInputPorts=2
  Scope1 : Scope
  Sum : Sum  Inputs=|++
  Sum1 : Sum  Inputs=|++
  Fz : Outport
  wires:
  Constant1/1 -> Product1/1
  d_dt/1 -> Product1/2
  Constant/1 -> Product/2
  Product1/1 -> Scope/2, Sum/2
  d/1 -> Sum1/1
  Product/1 -> Scope/1, Sum/1
  Sum/1 -> Scope1/1, Saturation/1
  Saturation/1 -> Fz/1
  Sum1/1 -> Saturation1/1
  Constant2/1 -> Sum1/2
  Saturation1/1 -> Product/1

== system UNIFIER/C7A_HARW/Subsystems/LandingGears/Nose/GearForceSystem/groundContactLogic3 ==
  in : Inport
  in_dt : Inport  Port=2
  flag : Inport  Port=3  OutDataTypeStr=boolean
  Constant : Constant  Value=0
  Switch : Switch  Criteria=u2 ~= 0  SaturateOnIntegerOverflow=off  InputSameDT=off
  Switch1 : Switch  Criteria=u2 > Threshold  SaturateOnIntegerOverflow=off  InputSameDT=off
  out : Outport
  out_dt : Outport  Port=2
  wires:
  Switch1/1 -> out_dt/1
  Switch/1 -> out/1
  in/1 -> Switch/1
  in_dt/1 -> Switch1/1
  flag/1 -> Switch1/2, Switch/2
  Constant/1 -> Switch/3, Switch1/3

== system UNIFIER/C7A_HARW/Subsystems/LandingGears/RightMain/DetermineGroundImpact/impactDetection ==
  note: Impact
  note: No impact
  X_tip : Inport
  ground_alt : Inport  Port=2
  Constant : Constant  OutDataTypeStr=boolean
  Constant1 : Constant  Value=0  OutDataTypeStr=boolean
  Selector1 : Selector  InputPortWidth=3  IndexOptions=Index vector (dialog)  Indices=3  OutputSizes=1
  Sum : Sum  Inputs=-+|
  Switch : Switch  Criteria=u2 > Threshold  SaturateOnIntegerOverflow=off  InputSameDT=off
  impact_flag : Outport
  distance_to_ground : Outport  Port=2
  wires:
  Constant1/1 -> Switch/1
  ground_alt/1 -> Sum/2
  X_tip/1 -> Selector1/1
  Selector1/1 -> Sum/1
  Switch/1 -> impact_flag/1
  Constant/1 -> Switch/3
  Sum/1 -> distance_to_ground/1, Switch/2

== system UNIFIER/C7A_HARW/Subsystems/LandingGears/RightMain/GearForceSystem/Forcez ==
  d : Inport
  d_dt : Inport  Port=2
  Constant : Constant  Value=110000
  Constant1 : Constant  Value=7000
  Constant2 : Constant  Value=0.15
  Product : Product
  Product1 : Product
  Saturation : Saturate  UpperLimit=0  LowerLimit=-inf
  Saturation1 : Saturate  UpperLimit=0  LowerLimit=-inf
  Scope : Scope  NumInputPorts=2
  Scope1 : Scope
  Sum : Sum  Inputs=|++
  Sum1 : Sum  Inputs=|++
  Fz : Outport
  wires:
  Constant1/1 -> Product1/1
  d_dt/1 -> Product1/2
  Constant/1 -> Product/2
  Product1/1 -> Scope/2, Sum/2
  d/1 -> Sum1/1
  Product/1 -> Scope/1, Sum/1
  Sum/1 -> Scope1/1, Saturation/1
  Saturation/1 -> Fz/1
  Sum1/1 -> Saturation1/1
  Constant2/1 -> Sum1/2
  Saturation1/1 -> Product/1

== system UNIFIER/C7A_HARW/Subsystems/LandingGears/RightMain/GearForceSystem/groundContactLogic3 ==
  in : Inport
  in_dt : Inport  Port=2
  flag : Inport  Port=3  OutDataTypeStr=boolean
  Constant : Constant  Value=0
  Switch : Switch  Criteria=u2 ~= 0  SaturateOnIntegerOverflow=off  InputSameDT=off
  Switch1 : Switch  Criteria=u2 > Threshold  SaturateOnIntegerOverflow=off  InputSameDT=off
  out : Outport
  out_dt : Outport  Port=2
  wires:
  Switch1/1 -> out_dt/1
  Switch/1 -> out/1
  in/1 -> Switch/1
  in_dt/1 -> Switch1/1
  flag/1 -> Switch1/2, Switch/2
  Constant/1 -> Switch/3, Switch1/3

== system UNIFIER/C7A_HARW/Subsystems/LandingGears/SideForceAndSteeringAndBraking/ForceSystem/MainGearBrake ==
  brake : Inport
  Fz_main : Inport  Port=2
  Abs2 : Abs  SaturateOnIntegerOverflow=off
  Constant1 : Constant  Value=-10000
  FrictionCoefficient : Gain  Gain=0.7
  Product1 : Product
  Saturation Dynamic : simulink/Discontinuities/Saturation Dynamic  OutMin=[]  OutMax=[]  OutDataTypeStr=Inherit: Same as second input  OutDataType=fixdt(1, 16)  OutScaling=2^-10  DoSatur=off
  Unary Minus1 : UnaryMinus
  Fx : Outport
  wires:
  Constant1/1 -> Product1/1
  brake/1 -> Product1/2
  Product1/1 -> Saturation Dynamic/2
  Unary Minus1/1 -> Saturation Dynamic/3
  FrictionCoefficient/1 -> Saturation Dynamic/1, Unary Minus1/1
  Abs2/1 -> FrictionCoefficient/1
  Saturation Dynamic/1 -> Fx/1
  Fz_main/1 -> Abs2/1

== system UNIFIER/C7A_HARW/Subsystems/LandingGears/SideForceAndSteeringAndBraking/ForceSystem/MainGearSideForce ==
  d_dt : Inport
  Fz_main : Inport  Port=2
  Abs2 : Abs  SaturateOnIntegerOverflow=off
  Constant1 : Constant  Value=150000
  FrictionCoefficient : Gain  Gain=0.7
  Product1 : Product
  Saturation Dynamic : simulink/Discontinuities/Saturation Dynamic  OutMin=[]  OutMax=[]  OutDataTypeStr=Inherit: Same as second input  OutDataType=fixdt(1, 16)  OutScaling=2^-10  DoSatur=off
  Unary Minus1 : UnaryMinus
  Fy : Outport
  wires:
  Constant1/1 -> Product1/1
  d_dt/1 -> Product1/2
  Product1/1 -> Saturation Dynamic/2
  Unary Minus1/1 -> Saturation Dynamic/3
  FrictionCoefficient/1 -> Saturation Dynamic/1, Unary Minus1/1
  Abs2/1 -> FrictionCoefficient/1
  Saturation Dynamic/1 -> Fy/1
  Fz_main/1 -> Abs2/1

== system UNIFIER/C7A_HARW/Subsystems/LandingGears/SideForceAndSteeringAndBraking/ForceSystem/NoseWheelSteer ==
  yaw_raw : Inport
  impact_flag_nose : Inport  Port=2
  Fz_nose : Inport  Port=3
  Abs2 : Abs  SaturateOnIntegerOverflow=off
  Constant1 : Constant  Value=0
  FrictionCoefficient : Gain  Gain=0.7
  Gain : Gain  Gain=4000
  Saturation Dynamic : simulink/Discontinuities/Saturation Dynamic  OutMin=[]  OutMax=[]  OutDataTypeStr=Inherit: Same as second input  OutDataType=fixdt(1, 16)  OutScaling=2^-10  DoSatur=off
  Switch : Switch  Criteria=u2 > Threshold  SaturateOnIntegerOverflow=off  InputSameDT=off
  Unary Minus1 : UnaryMinus
  y : Outport
  wires:
  FrictionCoefficient/1 -> Saturation Dynamic/1, Unary Minus1/1
  Fz_nose/1 -> Abs2/1
  Constant1/1 -> Switch/3
  Unary Minus1/1 -> Saturation Dynamic/3
  Saturation Dynamic/1 -> y/1
  Abs2/1 -> FrictionCoefficient/1
  Gain/1 -> Switch/1
  Switch/1 -> Saturation Dynamic/2
  yaw_raw/1 -> Gain/1
  impact_flag_nose/1 -> Switch/2

== system UNIFIER/C7A_HARW/Subsystems/LandingGears/SideForceAndSteeringAndBraking/ForceSystem/groundContactLogic3 ==
  in_dt : Inport
  flag : Inport  Port=2  OutDataTypeStr=boolean
  Constant : Constant  Value=0
  Switch1 : Switch  Criteria=u2 > Threshold  SaturateOnIntegerOverflow=off  InputSameDT=off
  out_dt : Outport
  wires:
  Switch1/1 -> out_dt/1
  in_dt/1 -> Switch1/1
  flag/1 -> Switch1/2
  Constant/1 -> Switch1/3

== matlab function UNIFIER/C7A_HARW/Subsystems/LandingGears/Nose/DetermineGroundImpact/MATLAB Function ==
  data: X_tip_in input size=3; impact_flag input; X_tip_memory input size=3; X_tip_out output size=3; X_tip_memory output
function [X_tip_out, X_tip_memory] = fcn(X_tip_in, impact_flag, X_tip_memory)

if impact_flag == true
    X_tip_out = X_tip_memory;
else
    X_tip_memory = X_tip_in;
    X_tip_out = X_tip_in;
end

== matlab function UNIFIER/X_PLANE_VISUALS/Subsystem4/DREF ==
  data: str input uint8; uint8_out output; value input single
function uint8_out = DREF_uint8(str, value)
% 1:5 = header
% 6:9 = value
% 10:x = dref_str
% x+1:509 = 0;

% Allocate:
uint8_out = uint8(' ' * ones(1,509));

% Packet:
uint8_out(1:5) = uint8('DREF0');
uint8_out(6:9) = typecast(value,'uint8');
uint8_out(10: 10 + numel(str) - 1) = str;
uint8_out(10 + numel(str)) = uint8(0);

== matlab function UNIFIER/X_PLANE_VISUALS/Subsystem5/DREF ==
  data: str input uint8; uint8_out output; value input single
function uint8_out = DREF_uint8(str, value)
% 1:5 = header
% 6:9 = value
% 10:x = dref_str
% x+1:509 = 0;

% Allocate:
uint8_out = uint8(' ' * ones(1,509));

% Packet:
uint8_out(1:5) = uint8('DREF0');
uint8_out(6:9) = typecast(value,'uint8');
uint8_out(10: 10 + numel(str) - 1) = str;
uint8_out(10 + numel(str)) = uint8(0);

== matlab function UNIFIER/X_PLANE_VISUALS/Subsystem6/DREF ==
  data: str input uint8; uint8_out output; value input single
function uint8_out = DREF_uint8(str, value)
% 1:5 = header
% 6:9 = value
% 10:x = dref_str
% x+1:509 = 0;

% Allocate:
uint8_out = uint8(' ' * ones(1,509));

% Packet:
uint8_out(1:5) = uint8('DREF0');
uint8_out(6:9) = typecast(value,'uint8');
uint8_out(10: 10 + numel(str) - 1) = str;
uint8_out(10 + numel(str)) = uint8(0);

== matlab function UNIFIER/X_PLANE_VISUALS/Subsystem7/DREF ==
  data: str input uint8; uint8_out output; value input single
function uint8_out = DREF_uint8(str, value)
% 1:5 = header
% 6:9 = value
% 10:x = dref_str
% x+1:509 = 0;

% Allocate:
uint8_out = uint8(' ' * ones(1,509));

% Packet:
uint8_out(1:5) = uint8('DREF0');
uint8_out(6:9) = typecast(value,'uint8');
uint8_out(10: 10 + numel(str) - 1) = str;
uint8_out(10 + numel(str)) = uint8(0);

== matlab function UNIFIER/X_PLANE_VISUALS/Subsystem8/DREF ==
  data: str input uint8; uint8_out output; value input single
function uint8_out = DREF_uint8(str, value)
% 1:5 = header
% 6:9 = value
% 10:x = dref_str
% x+1:509 = 0;

% Allocate:
uint8_out = uint8(' ' * ones(1,509));

% Packet:
uint8_out(1:5) = uint8('DREF0');
uint8_out(6:9) = typecast(value,'uint8');
uint8_out(10: 10 + numel(str) - 1) = str;
uint8_out(10 + numel(str)) = uint8(0);

== matlab function UNIFIER/X_PLANE_VISUALS/Subsystem9/DREF ==
  data: str input uint8; uint8_out output; value input single
function uint8_out = DREF_uint8(str, value)
% 1:5 = header
% 6:9 = value
% 10:x = dref_str
% x+1:509 = 0;

% Allocate:
uint8_out = uint8(' ' * ones(1,509));

% Packet:
uint8_out(1:5) = uint8('DREF0');
uint8_out(6:9) = typecast(value,'uint8');
uint8_out(10: 10 + numel(str) - 1) = str;
uint8_out(10 + numel(str)) = uint8(0);

== matlab function UNIFIER/X_PLANE_VISUALS/Subsystem10/DREF ==
  data: str input uint8; uint8_out output; value input single
function uint8_out = DREF_uint8(str, value)
% 1:5 = header
% 6:9 = value
% 10:x = dref_str
% x+1:509 = 0;

% Allocate:
uint8_out = uint8(' ' * ones(1,509));

% Packet:
uint8_out(1:5) = uint8('DREF0');
uint8_out(6:9) = typecast(value,'uint8');
uint8_out(10: 10 + numel(str) - 1) = str;
uint8_out(10 + numel(str)) = uint8(0);

== matlab function UNIFIER/X_PLANE_VISUALS/Subsystem11/DREF ==
  data: str input uint8; uint8_out output; value input single
function uint8_out = DREF_uint8(str, value)
% 1:5 = header
% 6:9 = value
% 10:x = dref_str
% x+1:509 = 0;

% Allocate:
uint8_out = uint8(' ' * ones(1,509));

% Packet:
uint8_out(1:5) = uint8('DREF0');
uint8_out(6:9) = typecast(value,'uint8');
uint8_out(10: 10 + numel(str) - 1) = str;
uint8_out(10 + numel(str)) = uint8(0);

== matlab function UNIFIER/X_PLANE_VISUALS/VEHA2 ==
  data: lat input double; uint8_out output; lon input double; h input double; psi input single; the input single; phi input single
function uint8_out = VEHX_uint8(lat, lon, h, psi, the, phi)
% 1:5 = header
% 6:9 = 0
% 10:17 = lat
% 18:25 = long
% 26:33 = h
% 34:37 = psi
% 38:41 = the
% 42:45 = phi

% Allocate:
uint8_out = uint8(zeros(1,45));

uint8_out(1:5) = uint8('VEHX0');

uint8_out(10:17) = typecast(lat,'uint8');
uint8_out(18:25) = typecast(lon,'uint8');
uint8_out(26:33) = typecast(h,'uint8');
uint8_out(34:37) = typecast(psi,'uint8');
uint8_out(38:41) = typecast(the,'uint8');
uint8_out(42:45) = typecast(phi,'uint8');

== matlab function UNIFIER/X_PLANE_VISUALS/Subsystem/DREF ==
  data: str input uint8; uint8_out output; value input single
function uint8_out = DREF_uint8(str, value)
% 1:5 = header
% 6:9 = value
% 10:x = dref_str
% x+1:509 = 0;

% Allocate:
uint8_out = uint8(' ' * ones(1,509));

% Packet:
uint8_out(1:5) = uint8('DREF0');
uint8_out(6:9) = typecast(value,'uint8');
uint8_out(10: 10 + numel(str) - 1) = str;
uint8_out(10 + numel(str)) = uint8(0);

== matlab function UNIFIER/X_PLANE_VISUALS/override_flightcontrol /Subsystem/DREF ==
  data: str input uint8; uint8_out output; value input single
function uint8_out = DREF_uint8(str, value)
% 1:5 = header
% 6:9 = value
% 10:x = dref_str
% x+1:509 = 0;

% Allocate:
uint8_out = uint8(' ' * ones(1,509));

% Packet:
uint8_out(1:5) = uint8('DREF0');
uint8_out(6:9) = typecast(value,'uint8');
uint8_out(10: 10 + numel(str) - 1) = str;
uint8_out(10 + numel(str)) = uint8(0);

== matlab function UNIFIER/C7A_HARW/Subsystems/LandingGears/RightMain/DetermineGroundImpact/MATLAB Function ==
  data: X_tip_in input size=3; impact_flag input; X_tip_memory input size=3; X_tip_out output size=3; X_tip_memory output
function [X_tip_out, X_tip_memory] = fcn(X_tip_in, impact_flag, X_tip_memory)

if impact_flag == true
    X_tip_out = X_tip_memory;
else
    X_tip_memory = X_tip_in;
    X_tip_out = X_tip_in;
end

== matlab function UNIFIER/X_PLANE_VISUALS/Subsystem1/DREF ==
  data: str input uint8; uint8_out output; value input single
function uint8_out = DREF_uint8(str, value)
% 1:5 = header
% 6:9 = value
% 10:x = dref_str
% x+1:509 = 0;

% Allocate:
uint8_out = uint8(' ' * ones(1,509));

% Packet:
uint8_out(1:5) = uint8('DREF0');
uint8_out(6:9) = typecast(value,'uint8');
uint8_out(10: 10 + numel(str) - 1) = str;
uint8_out(10 + numel(str)) = uint8(0);

== matlab function UNIFIER/X_PLANE_VISUALS/Subsystem2/DREF ==
  data: str input uint8; uint8_out output; value input single
function uint8_out = DREF_uint8(str, value)
% 1:5 = header
% 6:9 = value
% 10:x = dref_str
% x+1:509 = 0;

% Allocate:
uint8_out = uint8(' ' * ones(1,509));

% Packet:
uint8_out(1:5) = uint8('DREF0');
uint8_out(6:9) = typecast(value,'uint8');
uint8_out(10: 10 + numel(str) - 1) = str;
uint8_out(10 + numel(str)) = uint8(0);

== matlab function UNIFIER/X_PLANE_VISUALS/override_flightcontrol 1/Subsystem/DREF ==
  data: str input uint8; uint8_out output; value input single
function uint8_out = DREF_uint8(str, value)
% 1:5 = header
% 6:9 = value
% 10:x = dref_str
% x+1:509 = 0;

% Allocate:
uint8_out = uint8(' ' * ones(1,509));

% Packet:
uint8_out(1:5) = uint8('DREF0');
uint8_out(6:9) = typecast(value,'uint8');
uint8_out(10: 10 + numel(str) - 1) = str;
uint8_out(10 + numel(str)) = uint8(0);

== matlab function UNIFIER/X_PLANE_VISUALS/Subsystem3/DREF ==
  data: str input uint8; uint8_out output; value input single
function uint8_out = DREF_uint8(str, value)
% 1:5 = header
% 6:9 = value
% 10:x = dref_str
% x+1:509 = 0;

% Allocate:
uint8_out = uint8(' ' * ones(1,509));

% Packet:
uint8_out(1:5) = uint8('DREF0');
uint8_out(6:9) = typecast(value,'uint8');
uint8_out(10: 10 + numel(str) - 1) = str;
uint8_out(10 + numel(str)) = uint8(0);

== matlab function UNIFIER/C7A_HARW/Subsystems/LandingGears/LeftMain/DetermineGroundImpact/MATLAB Function ==
  data: X_tip_in input size=3; impact_flag input; X_tip_memory input size=3; X_tip_out output size=3; X_tip_memory output
function [X_tip_out, X_tip_memory] = fcn(X_tip_in, impact_flag, X_tip_memory)

if impact_flag == true
    X_tip_out = X_tip_memory;
else
    X_tip_memory = X_tip_in;
    X_tip_out = X_tip_in;
end
